simulink model "think_lab_demo"  (R2025b)
settings: Solver=VariableStepAuto  StartTime=0.0  StopTime=300  RelTol=1e-3
model workspace (MAT data in the model file):
  e_stop = 0
undefined symbols (not defined in the file): sampleTime, scanAngles
libraries: mobileRoboticsLib x4, simulink x2, robotalgslib x2, robotmobilelib x1
settings Model: PacingRate=1000  Creator=M  LastModifiedBy=M

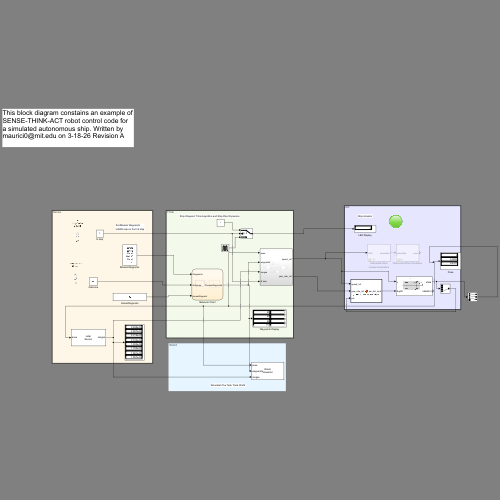
[thumbnail: Simulink's stored preview of the top-level diagram]
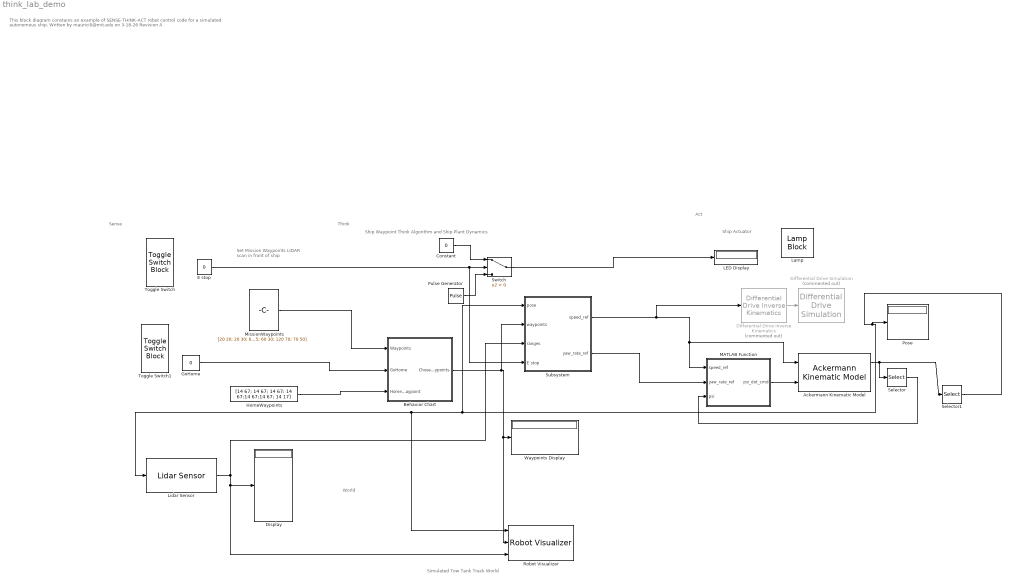
== system think_lab_demo ==
  note: Ship Waypoint Think Algorithm and Ship Plant Dynamics
  note: Set Mission Waypoints
      | LIDAR scan in front of ship
  note: Ship Actuator
  note: Simulated Tow Tank Track World
  note: This block diagram constains an example of SENSE-THINK-ACT robot control code for a simulated autonomous ship. Written by maurici0@mit.edu on 3-18-26 Revision A
  note: Act
  note: Think
  note: Sense
  note: World
  Ackermann Kinematic Model : robotmobilelib/Ackermann Kinematic Model  WheelBase=0.75  VehicleSpeedRange=[-0.5 0.5]  MaxSteeringAngle=2*pi/9  InitialState=[20; 20; 0.7; 0]  SimulateUsing=Interpreted execution
  Behavior Chart : Stateflow chart  TreatAsAtomicUnit=on
      settings: PortSchema="{\"entries\":[{\"content\":{\"sides\":[{\"content\":{\"connectorIds\":[\"In2\",\"In1\",\"In3\"]},\"type\":\"ConnectorPlacement.EquallySpacedRectSide\",\"uuid\":\"d8f81abb-7f32-4f84-af42-e6498a4032bf\"},{\"content\":{\"connectorIds\":[\"Out1\"],\"side\":\"RIGHT\"},\"type\":\"ConnectorPlacement.EquallySpacedRectSide\",\"uuid\":\"550ad4b0-fe8a-4be7-bef7-515b31a503dc\"},{\"content\":{\"side\":\"TOP\"},\"type\":\"ConnectorPlacement.EquallySpacedRectSide\",\"uuid\":\"65565bae-0b19-40d0-93e0-1df29585dffa\"}]},\"type\":\"ConnectorPlacement.EquallySpacedConnector\",\"uuid\":\"a86a927c-11e1-4724-81bd-5fb556ec99f6\"}],\"packageUris\":[\"http://schema.mathworks.com/mf0/Connector/R2020b\"],\"version\":\"1.0\"}"
  Constant : Constant  Value=0
  Differential Drive Inverse Kinematics : mobileRoboticsLib/Kinematic Models/Differential Drive/Differential Drive Inverse Kinematics  Commented=on  wheelRadius=R  wheelBase=L
      settings: SourceProductName=Mobile Robotics Simulation Toolbox
  Differential Drive Simulation : mobileRoboticsLib/Kinematic Models/Differential Drive/Differential Drive Simulation  Commented=on  wheelRadius=R  wheelBase=L  initX=20  initY=10  initAngle=0.7  Ts=sampleTime
      settings: SourceProductName=Mobile Robotics Simulation Toolbox
  Display : Display
  E stop : Constant  Value=0
  GoHome : Constant  Value=0
  HomeWaypoints : Constant  Value=[14 67; 14 67; 14 67; 14 67;14 67;14 67; 14 17]
  LED Display : Display
  Lamp : LampBlock  LabelPosition=Hide  DefaultColor=[192.0, 192.0, 192.0]
  Lidar Sensor : mobileRoboticsLib/Environments/Lidar Sensor  mapName=map2  sensorOffset=scanSensorOffset  scanAngles=scanAngles  maxRange=scanMaxRange
      settings: SourceProductName=Mobile Robotics Simulation Toolbox
  MATLAB Function : MATLAB Function  TreatAsAtomicUnit=on
  MissionWaypoints : Constant  Value=[20 20; 20 30; 60 30; 110 35; 60 30; 120 70; 70 50]
  Pose : Display
  Pulse Generator : DiscretePulseGenerator  PulseType=Time based  Period=10  PulseWidth=5
  Robot Visualizer : mobileRoboticsLib/Environments/Robot Visualizer  robotRadius=1  mapName=map2  showTrajectory=on  hasWaypoints=on  hasLidar=on  sensorOffset=scanSensorOffset  scanAngles=scanAngles  hasObjDetector=off  objDetectorOffset=[ 0, 0 ]  objDetectorAngle=0  objDetectorFOV=pi/4  objDetectorMaxRange=5  objectColors=[ 1, 0, 0; 0, 1, 0; 0, 0, 1 ]  objectMarkers=s
  Selector : Selector  InputPortWidth=4  IndexOptions=Index vector (dialog)  Indices=[4]  OutputSizes=1
  Selector1 : Selector  InputPortWidth=4  IndexOptions=Index vector (dialog)  Indices=[1 2 3]  OutputSizes=1
  Subsystem : Subsystem
  Switch : Switch  Criteria=u2 > Threshold  SaturateOnIntegerOverflow=off  InputSameDT=off
  Toggle Switch : ToggleSwitchBlock
  Toggle Switch1 : ToggleSwitchBlock
  Waypoints Display : Display
  wires:
  Constant/1 -> Switch/1
  Pulse Generator/1 -> Switch/3
  Switch/1 -> LED Display/1
  E stop/1 -> Subsystem/4(E stop), Switch/2
  MissionWaypoints/1 -> Behavior Chart/2(Waypoints)
  Differential Drive Inverse Kinematics/1 -> Differential Drive Simulation/1
  Selector1/1 -> Pose/1, Subsystem/1(pose), Robot Visualizer/1, Lidar Sensor/1
  Lidar Sensor/1 -> Robot Visualizer/3, Display/1, Subsystem/3(ranges)
  Subsystem/1(speed_ref) -> Ackermann Kinematic Model/1, MATLAB Function/1(speed_ref), Differential Drive Inverse Kinematics/1
  HomeWaypoints/1 -> Behavior Chart/3(HomeWaypoint)
  GoHome/1 -> Behavior Chart/1(GoHome)
  Behavior Chart/1(ChosenWaypoints) -> Subsystem/2(waypoints), Waypoints Display/1, Robot Visualizer/2
  Ackermann Kinematic Model/1 -> Selector1/1, Selector/1
  Selector/1 -> MATLAB Function/3(psi)
  Subsystem/2(yaw_rate_ref) -> MATLAB Function/2(yaw_rate_ref)
  MATLAB Function/1(psi_dot_cmd) -> Ackermann Kinematic Model/2

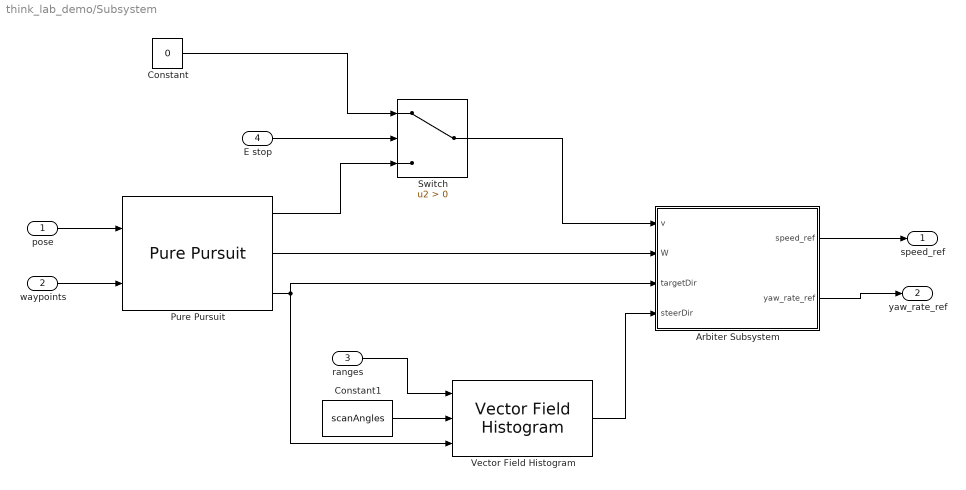
== system think_lab_demo/Subsystem ==
  pose : Inport
  waypoints : Inport  Port=2
  ranges : Inport  Port=3
  E stop : Inport  Port=4
  Arbiter Subsystem : Subsystem
  Constant : Constant  Value=0
  Constant1 : Constant  Value=scanAngles
  Pure Pursuit : robotalgslib/Pure Pursuit  DesiredLinearVelocityPort=off  DesiredLinearVelocity=1.5  MaxAngularVelocity=1.5  LookaheadDistancePort=off  LookaheadDistance=0.5  TargetDirPort=on  SimulateUsing=Interpreted execution
      settings: LibrarySourceBlock=navlib/Control Algorithms/Pure Pursuit
  Switch : Switch  Criteria=u2 > Threshold  SaturateOnIntegerOverflow=off  InputSameDT=off
  Vector Field Histogram : robotalgslib/Vector Field Histogram  NumAngularSectors=36  DistanceLimits=[ 0.05, 10 ]  HistogramThresholds=[ 5, 10 ]  RobotRadius=L  SafetyDistance=L  MinTurningRadius=0.25  SimulateUsing=Interpreted execution  TargetDirectionWeight=5  CurrentDirectionWeight=2  PreviousDirectionWeight=2
      settings: LibrarySourceBlock=navlib/Control Algorithms/Vector Field Histogram
  speed_ref : Outport
  yaw_rate_ref : Outport  Port=2
  wires:
  Arbiter Subsystem/1(speed_ref) -> speed_ref/1
  pose/1 -> Pure Pursuit/1
  waypoints/1 -> Pure Pursuit/2
  Constant/1 -> Switch/1
  E stop/1 -> Switch/2
  Pure Pursuit/1 -> Switch/3
  ranges/1 -> Vector Field Histogram/1
  Constant1/1 -> Vector Field Histogram/2
  Vector Field Histogram/1 -> Arbiter Subsystem/4(steerDir)
  Pure Pursuit/3 -> Vector Field Histogram/3, Arbiter Subsystem/3(targetDir)
  Pure Pursuit/2 -> Arbiter Subsystem/2(W)
  Switch/1 -> Arbiter Subsystem/1(v)
  Arbiter Subsystem/2(yaw_rate_ref) -> yaw_rate_ref/1

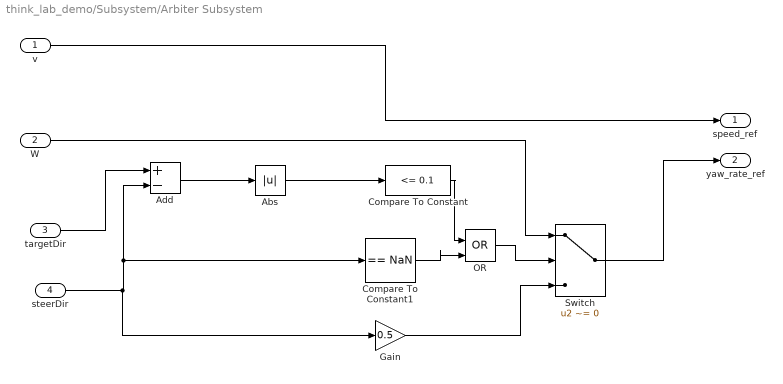
== system think_lab_demo/Subsystem/Arbiter Subsystem ==
  v : Inport
  W : Inport  Port=2
  targetDir : Inport  Port=3
  steerDir : Inport  Port=4
  Abs : Abs  SaturateOnIntegerOverflow=off
  Add : Sum  Inputs=+-
  Compare To Constant : simulink/Logic and Bit Operations/Compare To Constant  relop=<=  const=0.1  OutDataTypeStr=boolean
  Compare To Constant1 : simulink/Logic and Bit Operations/Compare To Constant  relop===  const=NaN  OutDataTypeStr=boolean
  Gain : Gain  Gain=0.5
  OR : Logic  Operator=OR  IconShape=distinctive  AllPortsSameDT=off  OutDataTypeStr=boolean
  Switch : Switch  Criteria=u2 ~= 0  SaturateOnIntegerOverflow=off  InputSameDT=off
  speed_ref : Outport
  yaw_rate_ref : Outport  Port=2
  wires:
  v/1 -> speed_ref/1
  Switch/1 -> yaw_rate_ref/1
  OR/1 -> Switch/2
  Gain/1 -> Switch/3
  W/1 -> Switch/1
  targetDir/1 -> Add/1
  steerDir/1 -> Gain/1, Add/2, Compare To Constant1/1
  Add/1 -> Abs/1
  Abs/1 -> Compare To Constant/1
  Compare To Constant/1 -> OR/1
  Compare To Constant1/1 -> OR/2

== matlab function think_lab_demo/MATLAB Function ==
  data: speed_ref input; psi_dot_cmd output; yaw_rate_ref input; psi input
function psi_dot_cmd = yawRateToSteeringRate(speed_ref, yaw_rate_ref, psi)
% Converts desired yaw rate into steering angle rate for Ackermann block.
%
% speed_ref: forward speed [m/s]
% yaw_rate_ref: desired yaw rate [rad/s]
% psi: current steering angle from Ackermann state output [rad]
%
% psi_dot_cmd: commanded steering angle rate [rad/s]

L = 0.75;   % effective wheelbase / turning length [m]
K = 6;      % steering response gain [1/s]

% Convert desired yaw rate into desired steering angle
if abs(speed_ref) < 1e-3
    psi_cmd = 0;
else
    psi_cmd = atan(L * yaw_rate_ref / speed_ref);
end

% Steering angle error
psi_error = psi_cmd - psi;

% Convert steering angle error into steering angular velocity
psi_dot_cmd = K * psi_error;

% Limit steering angular velocity, not steering angle
%psi_dot_max = 1.5; % rad/s
%psi_dot_cmd = min(max(psi_dot_cmd, -psi_dot_max), psi_dot_max);

end

== stateflow chart think_lab_demo/Behavior Chart ==
  state GoHome
    entry:
    ChosenWaypoints=HomeWaypoint
  state GoToWaypoint
    entry:
    ChosenWaypoints=Waypoints;
  note: Behavior-based finite state machine has just two states (more can easily be added later). Behavior state changes are initiated by monitoring GoHome external switch.
  (default) -> GoToWaypoint
  GoToWaypoint -> GoHome : [GoHome==1]
  GoHome -> GoToWaypoint : [GoHome==0]
  data: GoHome input; Waypoints input; HomeWaypoint input; ChosenWaypoints output
